simulink model "RL_TTS3_Controller_Blank_NLC"  (R2019b)
settings: Solver=FixedStepAuto  StartTime=0.0  StopTime=600  FixedStep=0.01  RelTol=1e-3
PostLoadFcn:
  | if any(exist('dsrtsu_mdlpostloadfcn', 'file') ~= 0), dsrtsu_mdlpostloadfcn('Execute', bdroot); end
libraries: simulink x2
settings Model: DSRTSU_INTERNAL_RTI_VER=550  DSRTSU_INTERNAL_RTI_TYPE=rti1104  RTICANMMDATA=struct('GeneralSetupData',struct('modelroot','E:\Will\RemoteLabs\TTS3\HostPC','generalsettings',struct('filesettings',struct('destfolder',struct('Name','RTICANMM_FILES','Check',1),'buildfolder',struct('Name','.','Check',1),'AbsDestfolder',struct('Name','E:\Will\RemoteLabs\TTS3\HostPC\RTICANMM_FILES'),'AbsBuildfolder',struct('Name','E:\Will\RemoteLabs\TTS3\HostPC'))),'options',struct('addpaths',1,'rmpaths',1,'addtrcexclusion',true,'cannavigator',struct('checkmonitoring',0),'show_usrtrc',0,'use_usrtrc',0),'advanced',struct('options',ones(1,100)),'MPSetup',{{}},'RTI',struct('Type','RTI1104','Ver','7.13','Date','02-Nov-2019'),'modelname','TTS3_Controller_Test_OL','block','TTS3_Controller_Test_OL'))  DSRTSU_INTERNAL_RTIFPGA=150  Creator=whendrix  LastModifiedBy=karan
settings OptimizationCC: BlockReduction=off  OptimizeBlockIOStorage=off  BufferReuse=off  GlobalBufferReuse=off  ExpressionFolding=off  LocalBlockOutputs=off  OptimizeDataStoreBuffers=off  BusAssignmentInplaceUpdate=off
settings DebuggingCC: BusObjectLabelMismatch=none
settings HardwareCC: ProdBitPerPointer=32  ProdBitPerSizeT=32  ProdBitPerPtrDiffT=32  ProdLargestAtomicInteger=Integer  ProdEndianess=BigEndian  ProdWordSize=32  ProdHWDeviceType=Custom Processor->Custom  TargetIntDivRoundTo=Zero  TargetEndianess=BigEndian  TargetHWDeviceType=Custom Processor->Custom
settings ModelReferenceCC: ModelReferenceNumInstancesAllowed=Single  ModelReferenceMinAlgLoopOccurrences=on
settings SFSimCC: MATLABDynamicMemAlloc=off  CustomCodeUndefinedFunction=UseInterfaceOnly
settings RTWCC: Description=dSPACE DS1104 Hardware Platform  SystemTargetFile=rti1104.tlc  MakeCommand=make_rti  TemplateMakefile=rti1104.tmf
settings CodeAppCC: MaxIdLength=63
settings STFCustomTargetCC: ParMdlRefBuildCompliant=on  SystemTargetFile=rti1104.tlc
settings GRTTargetCC: TargetLangStandard=C89/C90 (ANSI)  CompOptLevelCompliant=off  ConcurrentExecutionCompliant=off  CombineOutputUpdateFcns=off  MatFileLogging=off  CPPClassGenCompliant=off  UseToolchainInfoCompliant=off

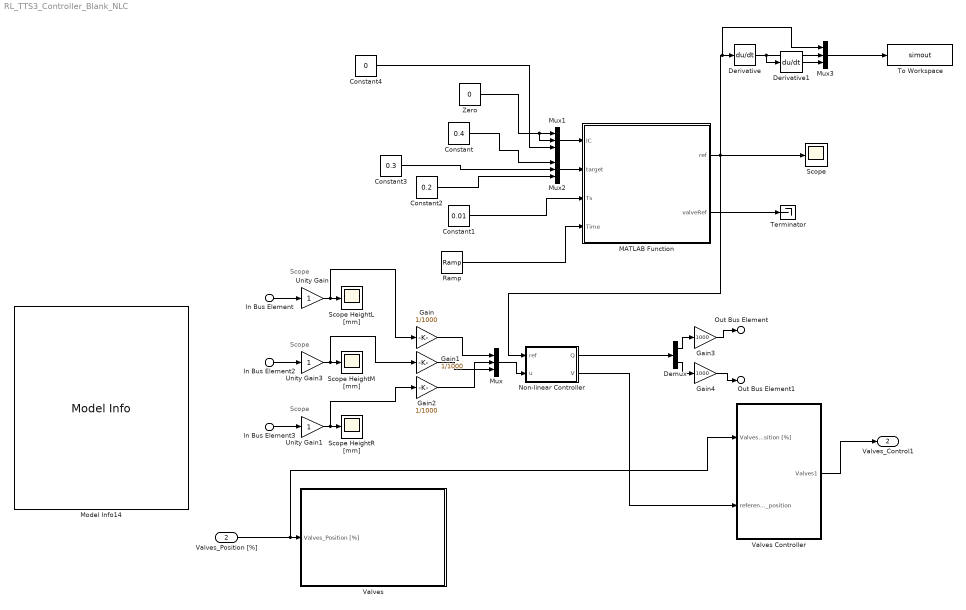
== system RL_TTS3_Controller_Blank_NLC ==
  note: Scope
  note: Scope
  note: Scope
  In Bus Element : Inport  PortName=Heights [mm]  Element=Left
  In Bus Element2 : Inport  PortName=Heights [mm]  Element=Middle
  In Bus Element3 : Inport  PortName=Heights [mm]  Element=Right
  Valves_Position [%] : Inport  Port=2  OutDataTypeStr=Bus: ValvesSOCI
  Constant : Constant  Value=0.4
  Constant1 : Constant  Value=0.01
  Constant2 : Constant  Value=0.2
  Constant3 : Constant  Value=0.3
  Constant4 : Constant  Value=0
  Demux : Demux  Outputs=2
  Derivative : Derivative
  Derivative1 : Derivative
  Gain : Gain  Gain=1/1000
  Gain1 : Gain  Gain=1/1000
  Gain2 : Gain  Gain=1/1000
  Gain3 : Gain  Gain=1000
  Gain4 : Gain  Gain=1000
  MATLAB Function : MATLAB Function  TreatAsAtomicUnit=on
  Model Info14 : simulink/Model-Wide Utilities/Model Info  Frame=on  DisplayStringWithTags=|  HorizontalTextAlignment=Left  LeftAlignmentValue=0.02
      | Start model for the "Three Tank"
      | experiment on the "Three Tank" setup.
      | Version: 1.0
      | 
      | 
      | INFORMATION
      | ----------------------
      | 
      | Unity Gain block before Scope is needed for
      | RemoteLabs compatebility. 
      | Do not modify or remove!
      | 
      | Pump range:
      | 0 to 0.102 [l/s]
      | 
      | The 5 Valves are labeled according 
      | to their position:
      | 
      |    LM  MR
      |      X     X
      |  X      X      X
      | LD    MD   RD
      | 
      | L = Left
      | M = Middle
      | R = Right
      | D = Down
  Mux{,1..3} (4 alike) : Mux  Inputs=3
  Non-linear Controller : MATLAB Function  TreatAsAtomicUnit=on
  Ramp : simulink/Sources/Ramp  slope=1  start=0  InitialOutput=0
  Scope : Scope
  Scope HeightL [mm] : Scope
  Scope HeightM [mm] : Scope
  Scope HeightR [mm] : Scope
  Terminator : Terminator
  To Workspace : ToWorkspace  VariableName=simout  SaveFormat=Timeseries  SampleTime=-1
  Unity Gain : Gain
  Unity Gain1 : Gain
  Unity Gain3 : Gain
  Valves : Subsystem  TreatAsAtomicUnit=on
  Valves Controller : Subsystem
  Zero : Constant  Value=0  OutDataTypeStr=Inherit: Inherit via back propagation
  Out Bus Element : Outport  VectorParamsAs1DForOutWhenUnconnected=off  PortName=Pumps [l/s]  Element=Left
  Out Bus Element1 : Outport  VectorParamsAs1DForOutWhenUnconnected=off  PortName=Pumps [l/s]  Element=Right
  Valves_Control1 : Outport  Port=2  OutDataTypeStr=Bus: ValvesSICO  VectorParamsAs1DForOutWhenUnconnected=off
  wires:
  Unity Gain/1 -> Gain/1, Scope HeightL [mm]/1
  Unity Gain3/1 -> Gain1/1, Scope HeightM [mm]/1
  Unity Gain1/1 -> Gain2/1, Scope HeightR [mm]/1
  In Bus Element/1 -> Unity Gain/1
  In Bus Element2/1 -> Unity Gain3/1
  In Bus Element3/1 -> Unity Gain1/1
  Valves_Position [%]/1 -> Valves Controller/1(Valves_Position [%]), Valves/1(Valves_Position [%])
  Mux/1 -> Non-linear Controller/2(u)
  Gain2/1 -> Mux/2
  Gain1/1 -> Mux/3
  Gain/1 -> Mux/1
  Non-linear Controller/1(Q) -> Demux/1
  Gain3/1 -> Out Bus Element/1
  Demux/1 -> Gain3/1
  Demux/2 -> Gain4/1
  Gain4/1 -> Out Bus Element1/1
  Valves Controller/1(Valves1) -> Valves_Control1/1
  Non-linear Controller/2(V) -> Valves Controller/2("reference_valve_position ")
  Mux1/1 -> MATLAB Function/1(IC)
  Mux3/1 -> To Workspace/1
  Constant/1 -> Mux2/1
  MATLAB Function/1(ref) -> Non-linear Controller/1(ref), Scope/1, Mux3/1, Derivative/1
  Constant4/1 -> Mux1/3
  MATLAB Function/2(valveRef) -> Terminator/1
  Constant3/1 -> Mux2/2
  Zero/1 -> Mux1/2, Mux1/1
  Derivative1/1 -> Mux3/3
  Constant1/1 -> MATLAB Function/3(Ts)
  Constant2/1 -> Mux2/3
  Derivative/1 -> Derivative1/1, Mux3/2
  Mux2/1 -> MATLAB Function/2(target)
  Ramp/1 -> MATLAB Function/4(Time)

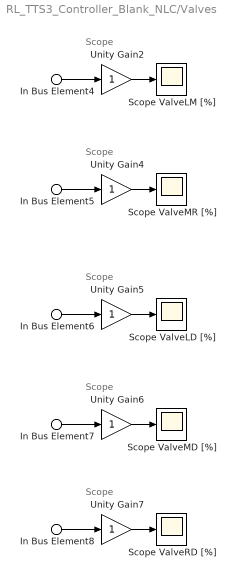
== system RL_TTS3_Controller_Blank_NLC/Valves ==
  note: Scope
  note: Scope
  note: Scope
  note: Scope
  note: Scope
  In Bus Element4 : Inport  PortName=Valves_Position [%]  Element=LeftMiddle
  In Bus Element5 : Inport  PortName=Valves_Position [%]  Element=MiddleRight
  In Bus Element6 : Inport  PortName=Valves_Position [%]  Element=LeftDown
  In Bus Element7 : Inport  PortName=Valves_Position [%]  Element=MiddleDown
  In Bus Element8 : Inport  PortName=Valves_Position [%]  Element=RightDown
  Scope ValveLD [%] : Scope
  Scope ValveLM [%] : Scope
  Scope ValveMD [%] : Scope
  Scope ValveMR [%] : Scope
  Scope ValveRD [%] : Scope
  Unity Gain{2,4..7} (5 alike) : Gain
  wires:
  In Bus Element5/1 -> Unity Gain4/1
  In Bus Element4/1 -> Unity Gain2/1
  In Bus Element7/1 -> Unity Gain6/1
  Unity Gain6/1 -> Scope ValveMD [%]/1
  In Bus Element6/1 -> Unity Gain5/1
  In Bus Element8/1 -> Unity Gain7/1
  Unity Gain7/1 -> Scope ValveRD [%]/1
  Unity Gain4/1 -> Scope ValveMR [%]/1
  Unity Gain5/1 -> Scope ValveLD [%]/1
  Unity Gain2/1 -> Scope ValveLM [%]/1

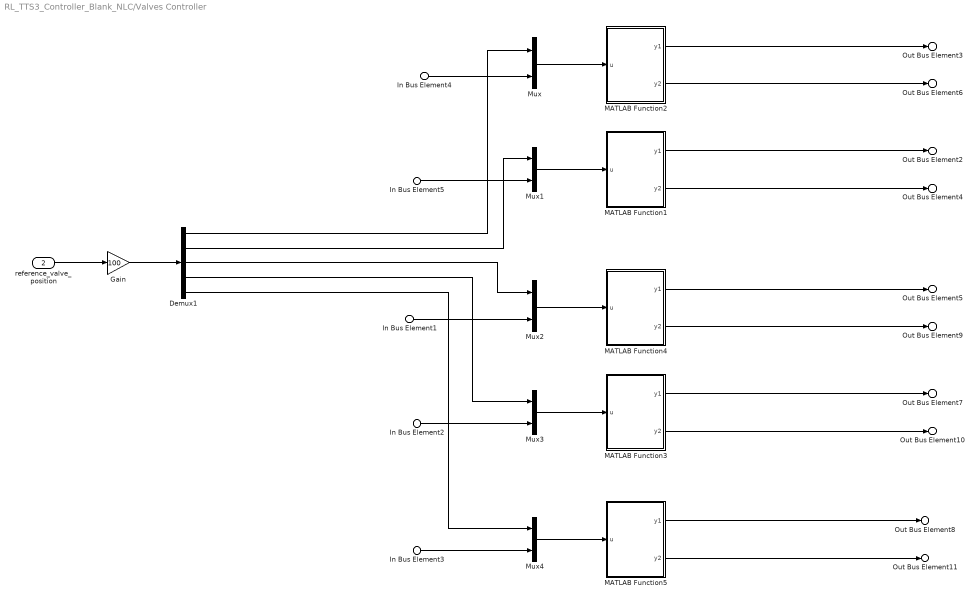
== system RL_TTS3_Controller_Blank_NLC/Valves Controller ==
  In Bus Element4 : Inport  PortName=Valves_Position [%]  Element=LeftMiddle
  In Bus Element5 : Inport  PortName=Valves_Position [%]  Element=MiddleRight
  In Bus Element1 : Inport  PortName=Valves_Position [%]  Element=LeftDown
  In Bus Element2 : Inport  PortName=Valves_Position [%]  Element=MiddleDown
  In Bus Element3 : Inport  PortName=Valves_Position [%]  Element=RightDown
  "reference_valve_position " : Inport  Port=2
  Demux1 : Demux  Outputs=5
  Gain : Gain  Gain=100
  MATLAB Function1 : MATLAB Function  TreatAsAtomicUnit=on
  MATLAB Function2 : MATLAB Function  TreatAsAtomicUnit=on
  MATLAB Function3 : MATLAB Function  TreatAsAtomicUnit=on
  MATLAB Function4 : MATLAB Function  TreatAsAtomicUnit=on
  MATLAB Function5 : MATLAB Function  TreatAsAtomicUnit=on
  Mux{,1..4} (5 alike) : Mux  Inputs=2
  Out Bus Element8 : Outport  VectorParamsAs1DForOutWhenUnconnected=off  PortName=Valves1  Element=RightDown.Open
  Out Bus Element11 : Outport  VectorParamsAs1DForOutWhenUnconnected=off  PortName=Valves1  Element=RightDown.Close
  Out Bus Element5 : Outport  VectorParamsAs1DForOutWhenUnconnected=off  PortName=Valves1  Element=LeftDown.Open
  Out Bus Element9 : Outport  VectorParamsAs1DForOutWhenUnconnected=off  PortName=Valves1  Element=LeftDown.Close
  Out Bus Element7 : Outport  VectorParamsAs1DForOutWhenUnconnected=off  PortName=Valves1  Element=MiddleDown.Open
  Out Bus Element10 : Outport  VectorParamsAs1DForOutWhenUnconnected=off  PortName=Valves1  Element=MiddleDown.Close
  Out Bus Element2 : Outport  VectorParamsAs1DForOutWhenUnconnected=off  PortName=Valves1  Element=MiddleRight.Open
  Out Bus Element4 : Outport  VectorParamsAs1DForOutWhenUnconnected=off  PortName=Valves1  Element=MiddleRight.Close
  Out Bus Element3 : Outport  VectorParamsAs1DForOutWhenUnconnected=off  PortName=Valves1  Element=LeftMiddle.Open
  Out Bus Element6 : Outport  VectorParamsAs1DForOutWhenUnconnected=off  PortName=Valves1  Element=LeftMiddle.Close
  wires:
  MATLAB Function4/1(y1) -> Out Bus Element5/1
  MATLAB Function4/2(y2) -> Out Bus Element9/1
  MATLAB Function5/1(y1) -> Out Bus Element8/1
  MATLAB Function5/2(y2) -> Out Bus Element11/1
  MATLAB Function3/2(y2) -> Out Bus Element10/1
  MATLAB Function3/1(y1) -> Out Bus Element7/1
  In Bus Element4/1 -> Mux/2
  Mux/1 -> MATLAB Function2/1(u)
  In Bus Element5/1 -> Mux1/2
  Demux1/2 -> Mux1/1
  MATLAB Function2/2(y2) -> Out Bus Element6/1
  MATLAB Function2/1(y1) -> Out Bus Element3/1
  Demux1/1 -> Mux/1
  Mux1/1 -> MATLAB Function1/1(u)
  MATLAB Function1/1(y1) -> Out Bus Element2/1
  MATLAB Function1/2(y2) -> Out Bus Element4/1
  Mux3/1 -> MATLAB Function3/1(u)
  Demux1/3 -> Mux2/1
  Demux1/4 -> Mux3/1
  In Bus Element2/1 -> Mux3/2
  Mux2/1 -> MATLAB Function4/1(u)
  In Bus Element1/1 -> Mux2/2
  In Bus Element3/1 -> Mux4/2
  Demux1/5 -> Mux4/1
  Mux4/1 -> MATLAB Function5/1(u)
  "reference_valve_position "/1 -> Gain/1
  Gain/1 -> Demux1/1

== matlab function RL_TTS3_Controller_Blank_NLC/Valves Controller/MATLAB Function2 ==
  data: u input; y1 output; y2 output
function [y1,y2] = fcn(u)
    if u(2)>u(1)
        y1 = false;
        y2 = true;
    elseif u(1)>u(2)
        y1 = true;
        y2 = false;
    else
        y1 = false;
        y2 = false;
    end
end

== matlab function RL_TTS3_Controller_Blank_NLC/Non-linear Controller ==
  data: ref input; u input; Q output; V output
function [Q,V] = fcn(ref,u)

x = [0 0 0];
% xr = [0.2 0.3 0.5];
xr = [ref(1) ref(2) ref(3)];
A = 0.0154; S = 5e-5; S_LM = .1; S_RM = .1; S_LD = 0.1; S_MD = 0.1; S_RD = 0.1; g = 9.81; 
x(1) = u(1);
x(2) = u(2);
x(3) = u(3);
Q = [0 0];
V = zeros(1,5);

Q1 = min(1.02e-4,A*(S_LD*S/A*sqrt(abs(2*g*x(1)))+S_LM*S/A*sqrt(2*g/abs(x(1)-x(3)))*(x(1)-x(3))-(x(1)-xr(1))));
Q2 = min(1.02e-4,A*(S_RD*S/A*sqrt(abs(2*g*x(2)))+S_RM*S/A*sqrt(2*g/abs(x(2)-x(3)))*(x(2)-x(3))-(x(2)-xr(2))));
if Q1<0
    Q1 = 0;
end
if Q2<0
    Q2=0;
end
Q(1) = Q1;
Q(2) = Q2;
V = [S_LM S_RM S_LD S_MD S_RD];

== matlab function RL_TTS3_Controller_Blank_NLC/Valves Controller/MATLAB Function1 ==
  data: u input; y1 output; y2 output
function [y1,y2] = fcn(u)
    if u(2)>u(1)
        y1 = false;
        y2 = true;
    elseif u(1)>u(2)
        y1 = true;
        y2 = false;
    else
        y1 = false;
        y2 = false;
    end
end

== matlab function RL_TTS3_Controller_Blank_NLC/Valves Controller/MATLAB Function3 ==
  data: u input; y1 output; y2 output
function [y1,y2] = fcn(u)
    if u(2)>u(1)
        y1 = false;
        y2 = true;
    elseif u(1)>u(2)
        y1 = true;
        y2 = false;
    else
        y1 = false;
        y2 = false;
    end
end

== matlab function RL_TTS3_Controller_Blank_NLC/Valves Controller/MATLAB Function4 ==
  data: u input; y1 output; y2 output
function [y1,y2] = fcn(u)
    if u(2)>u(1)
        y1 = false;
        y2 = true;
    elseif u(1)>u(2)
        y1 = true;
        y2 = false;
    else
        y1 = false;
        y2 = false;
    end
end

== matlab function RL_TTS3_Controller_Blank_NLC/Valves Controller/MATLAB Function5 ==
  data: u input; y1 output; y2 output
function [y1,y2] = fcn(u)
    if u(2)>u(1)
        y1 = false;
        y2 = true;
    elseif u(1)>u(2)
        y1 = true;
        y2 = false;
    else
        y1 = false;
        y2 = false;
    end
end

== matlab function RL_TTS3_Controller_Blank_NLC/MATLAB Function ==
  data: IC input; ref output; target input; valveRef output; Ts input; Time input
function [ref, valveRef] = fcn(IC, target,Ts,Time)
% input: IC, 3D vector of initial conditions of system
% input: target, 3D vector of target reference for fluid  heights
% input: Sampling time Ts

% output: ref, 3*1 vector containing fluid height references 
% output: valveRef, 2*1 vector containg valve references. Needed for MPC,
% can be ignored (use terminator block in simulink)

%% constants
Atank = 0.0154;
uMaxL = 0.1;        % from Bart's work
uMaxR =  0.09;      % from Bart's work
%% reshaping (check gode generation?)
IC = reshape(IC, [],1);             %  force IC to be a vector
target = reshape(target, [],1);     %  idem
%% calculations
tf = 1.1*sum(target)*Atank/(uMaxL+uMaxR-3*0.01)*1000;  % give a 10% margin for pump dynamics etc, choose 50% of maximum disturbance allowed as 'constant disturbance'
ref = zeros(3,1);
valveRef = zeros(2,1);
matr = [1 zeros(1,3);
        0 1  0    0;
        1 tf tf^2 tf^3;
        0 1 2*tf 3*tf^2];
invmatr = inv(matr);
if  Time < tf
    for i =1:3
        vec = [IC(i);0;target(i);0];
        polyCoeff = invmatr*vec;
        ref(i,1) = polyCoeff(1)+polyCoeff(2)*Time+polyCoeff(3)*Time.^2+polyCoeff(4)*Time.^3;
    end
else
    ref = target;
end
